simulink model "Prob3"  (R2020b)
settings: Solver=VariableStepAuto  StartTime=0.0  StopTime=10.0  RelTol=1e-3
undefined symbols (not defined in the file): b, m
settings Model: Creator=stkaravind  LastModifiedBy=stkaravind

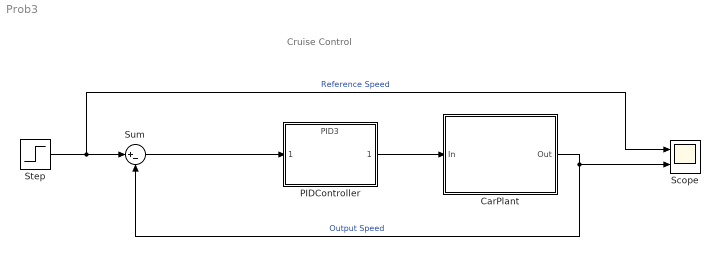
== system Prob3 ==
  note: Cruise Control
  CarPlant : Subsystem
  PIDController : ModelReference  ModelNameDialog=PID3  SimulationMode=Normal  ModelReferenceVersion=1.11
  Scope : Scope  NumInputPorts=2
  Step : Step  After=10  SampleTime=0
  Sum : Sum  Inputs=|+-
  wires:
  PIDController/1 -> CarPlant/1(In)
  Sum/1 -> PIDController/1
  CarPlant/1(Out) -> Scope/2, Sum/2  "Output Speed"
  Step/1 -> Scope/1, Sum/1  "Reference Speed"

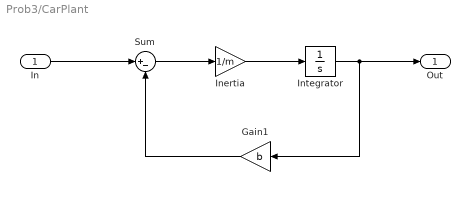
== system Prob3/CarPlant ==
  In : Inport
  Gain1 : Gain  Gain=b
  Inertia : Gain  Gain=1/m
  Integrator : Integrator
  Sum : Sum  Inputs=|+-
  Out : Outport
  wires:
  Inertia/1 -> Integrator/1
  Integrator/1 -> Out/1, Gain1/1
  Sum/1 -> Inertia/1
  Gain1/1 -> Sum/2
  In/1 -> Sum/1
